simulink model "behav_mcode_ckpt1_2021b_V2"  (R2021b)
settings: Solver=FixedStepDiscrete  StartTime=0.0  StopTime=40  FixedStep=1  RelTol=1e-3
(part 1 of 2)
settings Model: Creator=lisix  LastModifiedBy=lisixu
settings DebuggingCC: UnconnectedInputMsg=none  UnconnectedOutputMsg=none  UnconnectedLineMsg=none
settings RTWCC: DLArmComputeVersion=20.02.1

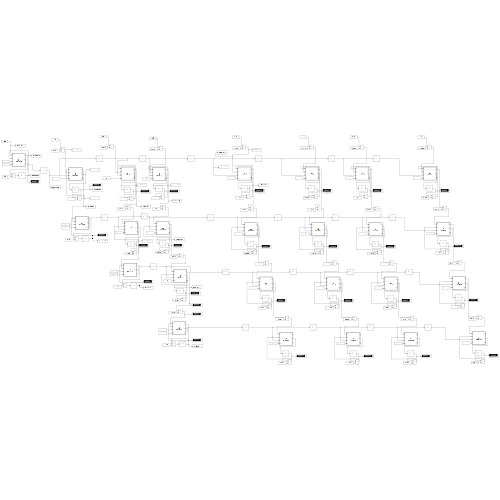
[thumbnail: Simulink's stored preview of the top-level diagram]
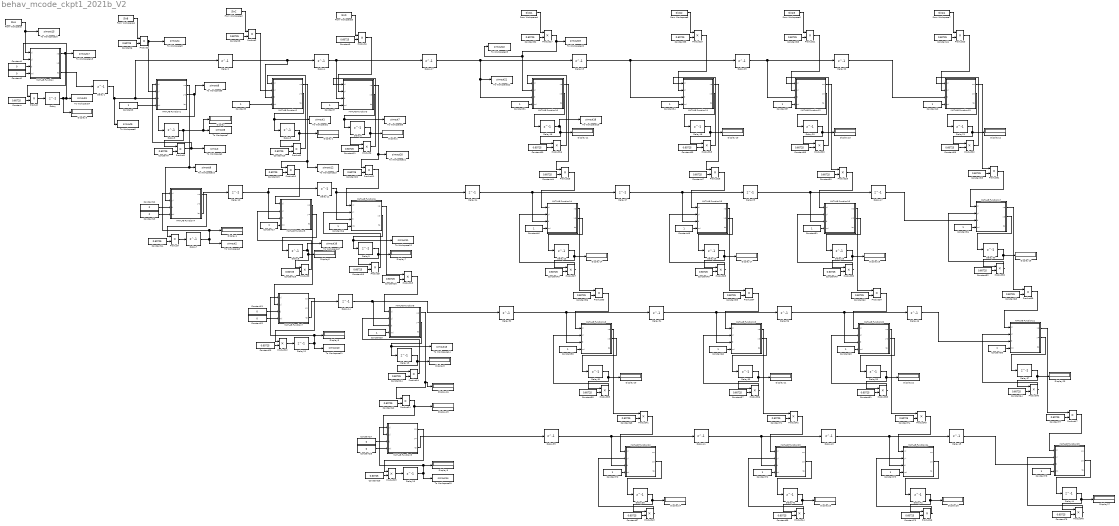
== system behav_mcode_ckpt1_2021b_V2 ==
  Constant{,4,6,8..11,14..15,18..20,23..24,26,29..30,32..33,35..36,38..39,41..45,47,49..50,52..53,55..57,59,61..62,64..65,67..69,71,73..74,76..77} (49 alike) : Constant  Value=0.60725
  Constant{1..2,12..13,21..22,27..28} (8 alike) : Constant  Value=0
  Constant{3,5,7,16..17,25,31,34,37,40,46,48,51,54,58,60,63,66,70,72,75,78} (22 alike) : Constant
  Delay{,1..47} (48 alike) : Delay  DelayLength=1  InitialCondition=0
  Display{,1..27} (28 alike) : Display
  From Workspace : FromWorkspace  VariableName=SlxA  OutputAfterFinalValue=Setting to zero
  From Workspace1 : FromWorkspace  VariableName=SlxB  OutputAfterFinalValue=Setting to zero
  From Workspace2 : FromWorkspace  VariableName=SlxC  OutputAfterFinalValue=Setting to zero
  From Workspace3 : FromWorkspace  VariableName=SlxD  OutputAfterFinalValue=Setting to zero
  From Workspace4 : FromWorkspace  VariableName=SlxQ1  OutputAfterFinalValue=Setting to zero
  From Workspace5 : FromWorkspace  VariableName=SlxQ2  OutputAfterFinalValue=Setting to zero
  From Workspace6 : FromWorkspace  VariableName=SlxQ3  OutputAfterFinalValue=Setting to zero
  From Workspace7 : FromWorkspace  VariableName=SlxQ4  OutputAfterFinalValue=Setting to zero
  MATLAB Function : MATLAB Function  TreatAsAtomicUnit=on
  MATLAB Function1 : MATLAB Function  TreatAsAtomicUnit=on
  MATLAB Function10 : MATLAB Function  TreatAsAtomicUnit=on
  MATLAB Function11 : MATLAB Function  TreatAsAtomicUnit=on
  MATLAB Function12 : MATLAB Function  TreatAsAtomicUnit=on
  MATLAB Function13 : MATLAB Function  TreatAsAtomicUnit=on
  MATLAB Function14 : MATLAB Function  TreatAsAtomicUnit=on
  MATLAB Function15 : MATLAB Function  TreatAsAtomicUnit=on
  MATLAB Function16 : MATLAB Function  TreatAsAtomicUnit=on
  MATLAB Function17 : MATLAB Function  TreatAsAtomicUnit=on
  MATLAB Function18 : MATLAB Function  TreatAsAtomicUnit=on
  MATLAB Function19 : MATLAB Function  TreatAsAtomicUnit=on
  MATLAB Function2 : MATLAB Function  TreatAsAtomicUnit=on
  MATLAB Function20 : MATLAB Function  TreatAsAtomicUnit=on
  MATLAB Function21 : MATLAB Function  TreatAsAtomicUnit=on
  MATLAB Function22 : MATLAB Function  TreatAsAtomicUnit=on
  MATLAB Function23 : MATLAB Function  TreatAsAtomicUnit=on
  MATLAB Function24 : MATLAB Function  TreatAsAtomicUnit=on
  MATLAB Function25 : MATLAB Function  TreatAsAtomicUnit=on
  MATLAB Function3 : MATLAB Function  TreatAsAtomicUnit=on
  MATLAB Function4 : MATLAB Function  TreatAsAtomicUnit=on
  MATLAB Function5 : MATLAB Function  TreatAsAtomicUnit=on
  MATLAB Function6 : MATLAB Function  TreatAsAtomicUnit=on
  MATLAB Function7 : MATLAB Function  TreatAsAtomicUnit=on
  MATLAB Function8 : MATLAB Function  TreatAsAtomicUnit=on
  MATLAB Function9 : MATLAB Function  TreatAsAtomicUnit=on
  Product{,1..48} (49 alike) : Product
  To Workspace1 : ToWorkspace  VariableName=simout1  SaveFormat=Timeseries  SampleTime=-1
  To Workspace10 : ToWorkspace  VariableName=simout9  SaveFormat=Timeseries  SampleTime=-1
  To Workspace11 : ToWorkspace  VariableName=simout10  SaveFormat=Timeseries  SampleTime=-1
  To Workspace12 : ToWorkspace  VariableName=simout11  SaveFormat=Timeseries  SampleTime=-1
  To Workspace13 : ToWorkspace  VariableName=simout12  SaveFormat=Timeseries  SampleTime=-1
  To Workspace14 : ToWorkspace  VariableName=simout13  SaveFormat=Timeseries  SampleTime=-1
  To Workspace15 : ToWorkspace  VariableName=simout14  SaveFormat=Timeseries  SampleTime=-1
  To Workspace16 : ToWorkspace  VariableName=simout15  SaveFormat=Timeseries  SampleTime=-1
  To Workspace17 : ToWorkspace  VariableName=simout16  SaveFormat=Timeseries  SampleTime=-1
  To Workspace18 : ToWorkspace  VariableName=simout17  SaveFormat=Timeseries  SampleTime=-1
  To Workspace19 : ToWorkspace  VariableName=simout18  SaveFormat=Timeseries  SampleTime=-1
  To Workspace2 : ToWorkspace  VariableName=simout  SaveFormat=Timeseries  SampleTime=-1
  To Workspace20 : ToWorkspace  VariableName=simout19  SaveFormat=Timeseries  SampleTime=-1
  To Workspace21 : ToWorkspace  VariableName=simout20  SaveFormat=Timeseries  SampleTime=-1
  To Workspace22 : ToWorkspace  VariableName=simout21  SaveFormat=Timeseries  SampleTime=-1
  To Workspace23 : ToWorkspace  VariableName=simout22  SaveFormat=Timeseries  SampleTime=-1
  To Workspace3 : ToWorkspace  VariableName=simout2  SaveFormat=Timeseries  SampleTime=-1
  To Workspace4 : ToWorkspace  VariableName=simout3  SaveFormat=Timeseries  SampleTime=-1
  To Workspace5 : ToWorkspace  VariableName=simout4  SaveFormat=Timeseries  SampleTime=-1
  To Workspace6 : ToWorkspace  VariableName=simout5  SaveFormat=Timeseries  SampleTime=-1
  To Workspace7 : ToWorkspace  VariableName=simout6  SaveFormat=Timeseries  SampleTime=-1
  To Workspace8 : ToWorkspace  VariableName=simout7  SaveFormat=Timeseries  SampleTime=-1
  To Workspace9 : ToWorkspace  VariableName=simout8  SaveFormat=Timeseries  SampleTime=-1
  wires:
  MATLAB Function/1(xo) -> To Workspace18/1, Product/1
  Product/1 -> Delay/1
  Delay/1 -> Display3/1, MATLAB Function/2(yi), To Workspace4/1
  Constant/1 -> Product/2
  Constant1/1 -> MATLAB Function/3(ti)
  Constant2/1 -> MATLAB Function/4(mi)
  MATLAB Function/3(to) -> Delay1/1
  Constant3/1 -> MATLAB Function1/4(mi)
  Delay1/1 -> To Workspace6/1, Delay2/1, MATLAB Function1/3(ti)
  From Workspace1/1 -> Product3/1
  Delay3/1 -> Display/1, To Workspace7/1, Product1/1
  Constant6/1 -> Product3/2
  Constant4/1 -> Product1/2
  Product1/1 -> MATLAB Function1/1(xi), To Workspace2/1
  Delay2/1 -> Delay4/1, MATLAB Function2/3(ti)
  Constant5/1 -> MATLAB Function2/4(mi)
  Constant7/1 -> MATLAB Function3/4(mi)
  Delay4/1 -> Delay17/1, MATLAB Function3/3(ti)
  Constant8/1 -> Product2/2
  From Workspace2/1 -> Product2/1
  Product2/1 -> MATLAB Function2/2(yi)
  Constant9/1 -> Product4/2
  From Workspace3/1 -> Product4/1
  Product4/1 -> MATLAB Function3/2(yi)
  Constant10/1 -> Product5/2
  Delay5/1 -> Display1/1, Product5/1
  Product5/1 -> MATLAB Function2/1(xi)
  Constant11/1 -> Product6/2
  Delay6/1 -> Display2/1, Product6/1
  Product6/1 -> MATLAB Function3/1(xi)
  Product3/1 -> MATLAB Function1/2(yi), To Workspace5/1
  From Workspace/1 -> To Workspace16/1, MATLAB Function/1(xi)
  MATLAB Function1/2(yo) -> Delay3/1, To Workspace9/1
  MATLAB Function2/2(yo) -> To Workspace1/1, Delay5/1
  MATLAB Function3/2(yo) -> To Workspace8/1, Delay6/1
  Constant12/1 -> MATLAB Function4/3(ti)
  Constant13/1 -> MATLAB Function4/4(mi)
  Constant14/1 -> Product7/2
  Product7/1 -> Delay7/1
  Delay7/1 -> To Workspace3/1, Display4/1, MATLAB Function4/1(xi)
  MATLAB Function4/1(xo) -> Product7/1
  MATLAB Function1/1(xo) -> MATLAB Function4/2(yi), To Workspace10/1
  Constant16/1 -> MATLAB Function6/4(mi)
  Constant15/1 -> Product9/2
  MATLAB Function6/2(yo) -> To Workspace12/1, Delay9/1
  Delay8/1 -> To Workspace17/1, Display6/1, Product8/1
  Delay9/1 -> Display7/1, Product9/1
  MATLAB Function4/3(to) -> Delay10/1
  Delay10/1 -> Delay11/1, MATLAB Function5/3(ti)
  Constant17/1 -> MATLAB Function5/4(mi)
  Delay11/1 -> Delay24/1, MATLAB Function6/3(ti)
  MATLAB Function3/1(xo) -> To Workspace21/1, Product11/1
  Constant18/1 -> Product8/2
  MATLAB Function2/1(xo) -> Product10/1, To Workspace13/1
  Constant19/1 -> Product10/2
  MATLAB Function5/2(yo) -> Delay8/1
  Constant20/1 -> Product11/2
  Product9/1 -> MATLAB Function6/2(yi)
  Product10/1 -> MATLAB Function5/1(xi)
  Product8/1 -> MATLAB Function5/2(yi)
  Constant23/1 -> Product12/2
  Constant21/1 -> MATLAB Function7/3(ti)
  Product12/1 -> Delay12/1
  Delay12/1 -> Display5/1, MATLAB Function7/1(xi), To Workspace11/1
  MATLAB Function7/1(xo) -> Product12/1
  Constant22/1 -> MATLAB Function7/4(mi)
  MATLAB Function5/1(xo) -> MATLAB Function7/2(yi)
  Delay13/1 -> Display8/1, Product14/1
  MATLAB Function8/2(yo) -> To Workspace14/1, Delay13/1
  Constant24/1 -> Product14/2
  Constant25/1 -> MATLAB Function8/4(mi)
  Product14/1 -> MATLAB Function8/2(yi)
  Constant26/1 -> Product13/2
  MATLAB Function6/1(xo) -> Product13/1
  Product13/1 -> MATLAB Function8/1(xi)
  Product11/1 -> MATLAB Function6/1(xi)
  MATLAB Function7/3(to) -> Delay14/1
  MATLAB Function9/1(xo) -> Product15/1
  Constant27/1 -> MATLAB Function9/3(ti)
  Constant28/1 -> MATLAB Function9/4(mi)
  Constant29/1 -> Product15/2
  Product15/1 -> Delay15/1
  Delay15/1 -> Display9/1, MATLAB Function9/1(xi), To Workspace15/1
  Constant31/1 -> MATLAB Function10/4(mi)
  MATLAB Function10/2(yo) -> Delay16/1
  Delay16/1 -> To Workspace19/1, Display11/1, Product16/1
  Constant32/1 -> Product17/2
  From Workspace4/1 -> Product17/1
  Constant30/1 -> Product16/2
  From Workspace5/1 -> Product19/1
  Constant35/1 -> Product19/2
  Product19/1 -> MATLAB Function11/2(yi)
  Constant33/1 -> Product18/2
  Delay18/1 -> Display10/1, Product18/1
  Product18/1 -> MATLAB Function11/1(xi)
  Constant34/1 -> MATLAB Function11/4(mi)
  MATLAB Function11/2(yo) -> Delay18/1
  Delay17/1 -> Delay19/1, To Workspace22/1, MATLAB Function10/3(ti)
  From Workspace6/1 -> Product21/1
  Constant38/1 -> Product21/2
  Product21/1 -> MATLAB Function12/2(yi)
  Constant36/1 -> Product20/2
  Product23/1 -> MATLAB Function13/2(yi)
  Constant41/1 -> Product23/2
  From Workspace7/1 -> Product23/1
  Delay21/1 -> Display12/1, Product22/1
  Constant39/1 -> Product22/2
  Delay20/1 -> Display13/1, Product20/1
  Product20/1 -> MATLAB Function12/1(xi)
  MATLAB Function12/2(yo) -> Delay20/1
  Delay19/1 -> Delay25/1, MATLAB Function11/3(ti)
  MATLAB Function13/2(yo) -> Delay21/1
  Constant40/1 -> MATLAB Function13/4(mi)
  Constant37/1 -> MATLAB Function12/4(mi)
  Product22/1 -> MATLAB Function13/1(xi)
  Constant42/1 -> Product24/2
  Product24/1 -> Display15/1, MATLAB Function9/2(yi)
  Delay24/1 -> Delay27/1, MATLAB Function14/3(ti)
  Delay23/1 -> Display14/1, Product27/1
  MATLAB Function10/1(xo) -> Product25/1
  Constant43/1 -> Product27/2
  Constant46/1 -> MATLAB Function14/4(mi)
  Constant44/1 -> Product25/2
  Delay25/1 -> Delay22/1, MATLAB Function12/3(ti)
  MATLAB Function8/1(xo) -> Product24/1, Display16/1
  Delay22/1 -> MATLAB Function13/3(ti)
  Product27/1 -> MATLAB Function14/2(yi)
  Product25/1 -> MATLAB Function14/1(xi)
  MATLAB Function14/2(yo) -> Delay23/1
  Delay27/1 -> Delay29/1, MATLAB Function15/3(ti)
  Constant47/1 -> Product26/2
  Constant48/1 -> MATLAB Function15/4(mi)
  Constant45/1 -> Product28/2
  MATLAB Function11/1(xo) -> Product26/1
  MATLAB Function15/2(yo) -> Delay26/1
  Product28/1 -> MATLAB Function15/2(yi)
  Delay26/1 -> Display17/1, Product28/1
  Product26/1 -> MATLAB Function15/1(xi)
  MATLAB Function16/2(yo) -> Delay28/1
  Constant49/1 -> Product30/2
  MATLAB Function12/1(xo) -> Product29/1
  Product29/1 -> MATLAB Function16/1(xi)
  Constant51/1 -> MATLAB Function16/4(mi)
  Constant50/1 -> Product29/2
  Delay28/1 -> Display18/1, Product30/1
  Product30/1 -> MATLAB Function16/2(yi)
  Product31/1 -> MATLAB Function17/1(xi)
  Constant53/1 -> Product31/2
  Delay29/1 -> Delay47/1, MATLAB Function16/3(ti)
  Constant54/1 -> MATLAB Function17/4(mi)
  Delay30/1 -> Display19/1, Product32/1
  Constant52/1 -> Product32/2
  MATLAB Function13/1(xo) -> Product31/1
  Product32/1 -> MATLAB Function17/2(yi)
  MATLAB Function17/2(yo) -> Delay30/1
  Delay14/1 -> Delay32/1, MATLAB Function8/3(ti)
  Delay32/1 -> Delay34/1, MATLAB Function18/3(ti)
  MATLAB Function19/2(yo) -> Delay33/1
  Constant56/1 -> Product33/2
  Constant55/1 -> Product35/2
  MATLAB Function15/1(xo) -> Product34/1
  MATLAB Function18/2(yo) -> Delay31/1
  Constant66/1 -> MATLAB Function21/4(mi)
  Delay37/1 -> Display23/1, Product40/1
  Product40/1 -> MATLAB Function21/2(yi)
  Constant64/1 -> Product40/2
  Product34/1 -> MATLAB Function19/1(xi)
  Constant58/1 -> MATLAB Function18/4(mi)
  MATLAB Function21/2(yo) -> Delay37/1
  MATLAB Function14/1(xo) -> Product33/1
  Constant59/1 -> Product34/2
  Delay34/1 -> Delay36/1, MATLAB Function19/3(ti)
  Product33/1 -> MATLAB Function18/1(xi)
  Constant60/1 -> MATLAB Function19/4(mi)
  Delay31/1 -> Display20/1, Product35/1
  MATLAB Function17/1(xo) -> Product39/1
  Product35/1 -> MATLAB Function18/2(yi)
  Product38/1 -> MATLAB Function20/2(yi)
  Constant65/1 -> Product39/2
  Product37/1 -> MATLAB Function20/1(xi)
  Constant62/1 -> Product37/2
  Delay36/1 -> Delay46/1, MATLAB Function20/3(ti)
  Constant57/1 -> Product36/2
  Constant63/1 -> MATLAB Function20/4(mi)
  Constant61/1 -> Product38/2
  MATLAB Function16/1(xo) -> Product37/1
  MATLAB Function20/2(yo) -> Delay35/1
  Product36/1 -> MATLAB Function19/2(yi)
  Product39/1 -> MATLAB Function21/1(xi)
  Delay33/1 -> Display21/1, Product36/1
  Delay35/1 -> Display22/1, Product38/1
  MATLAB Function21/1(xo) -> Product47/1
  MATLAB Function25/2(yo) -> Delay44/1
  Product48/1 -> MATLAB Function25/2(yi)
  Constant78/1 -> MATLAB Function25/4(mi)
  MATLAB Function22/2(yo) -> Delay38/1
  Delay41/1 -> Delay43/1, MATLAB Function23/3(ti)
  Constant67/1 -> Product43/2
  Constant71/1 -> Product42/2
  Constant68/1 -> Product41/2
  MATLAB Function19/1(xo) -> Product42/1
  Constant73/1 -> Product46/2
  Constant69/1 -> Product44/2
  Delay39/1 -> Delay41/1, MATLAB Function22/3(ti)
  Constant75/1 -> MATLAB Function24/4(mi)
  Constant74/1 -> Product45/2
  Delay43/1 -> Delay45/1, MATLAB Function24/3(ti)
  Product42/1 -> MATLAB Function23/1(xi)
  Product43/1 -> MATLAB Function22/2(yi)
  Constant77/1 -> Product47/2
  Product46/1 -> MATLAB Function24/2(yi)
  Product45/1 -> MATLAB Function24/1(xi)
  Delay38/1 -> Display24/1, Product43/1
  Product41/1 -> MATLAB Function22/1(xi)
  MATLAB Function18/1(xo) -> Product41/1
  Constant72/1 -> MATLAB Function23/4(mi)
  Constant76/1 -> Product48/2
  Delay42/1 -> Display26/1, Product46/1
  Delay40/1 -> Display25/1, Product44/1
  Delay44/1 -> Display27/1, Product48/1
  Product44/1 -> MATLAB Function23/2(yi)
  MATLAB Function24/2(yo) -> Delay42/1
  MATLAB Function23/2(yo) -> Delay40/1
  MATLAB Function20/1(xo) -> Product45/1
  Product47/1 -> MATLAB Function25/1(xi)
  Constant70/1 -> MATLAB Function22/4(mi)
  MATLAB Function9/3(to) -> Delay39/1
  Product16/1 -> MATLAB Function10/1(xi)
  Product17/1 -> To Workspace20/1, MATLAB Function10/2(yi), To Workspace23/1
  Delay45/1 -> MATLAB Function25/3(ti)
  Delay46/1 -> MATLAB Function21/3(ti)
  Delay47/1 -> MATLAB Function17/3(ti)

== matlab function behav_mcode_ckpt1_2021b_V2/MATLAB Function8 ==
  data: xi input; xo output; yi input; ti input; mi input; yo output; to output
function [xo,yo,to] = cordicVanilla(xi,yi,ti,mi)
cordic_phase=[0.78539816339744828000,0.46364760900080609000,0.24497866312686414000,0.12435499454676144000,0.06241880999595735000,0.03123983343026827700,0.01562372862047683100,0.00781234106010111110,0.00390623013196697180,0.00195312251647881880,0.00097656218955931946,0.00048828121119489829,0.00024414062014936177,0.00012207031189367021,0.00006103515617420877,0.00003051757811552610,0.00001525878906131576,0.00000762939453110197,0.00000381469726560650,0.00000190734863281019,0.00000095367431640596,0.00000047683715820309,0.00000023841857910156,0.00000011920928955078,0.00000005960464477539,0.00000002980232238770,0.00000001490116119385,0.00000000745058059692,0.00000000372529029846,0.00000000186264514923,0.00000000093132257462,0.00000000046566128731,0.00000000023283064365,0.00000000011641532183,0.00000000005820766091,0.00000000002910383046,0.00000000001455191523,0.00000000000727595761,0.00000000000363797881,0.00000000000181898940,0.00000000000090949470,0.00000000000045474735,0.00000000000022737368,0.00000000000011368684,0.00000000000005684342,0.00000000000002842171,0.00000000000001421085,0.00000000000000710543,0.00000000000000355271,0.00000000000000177636,0.00000000000000088818,0.00000000000000044409,0.00000000000000022204,0.00000000000000011102,0.00000000000000005551,0.00000000000000002776,0.00000000000000001388,0.00000000000000000694,0.00000000000000000347,0.00000000000000000173,0.00000000000000000087,0.00000000000000000043,0.00000000000000000022,0.00000000000000000011];

x = xi;
y = yi;
t = 0;
if mi
    t = ti;
else
    t = 0;
end
for i = 1:1:20
    sigma = 0;
    if mi
        if t < 0
            sigma = -1;
        else
            sigma = 1;
        end
    else
        if y < 0
            sigma = 1;
        else
            sigma = -1;
        end
    end
    xs = x * sigma * 2^(-(i-1));
    ys = y * sigma * 2^(-(i-1));
    x = x - ys;
    y = y + xs;
    t = t - sigma * cordic_phase(i);
end
xo = x;
yo = y;
to = t;
end

== matlab function behav_mcode_ckpt1_2021b_V2/MATLAB Function1 ==
  data: xi input; xo output; yi input; ti input; mi input; yo output; to output
function [xo,yo,to] = cordicVanilla(xi,yi,ti,mi)
cordic_phase=[0.78539816339744828000,0.46364760900080609000,0.24497866312686414000,0.12435499454676144000,0.06241880999595735000,0.03123983343026827700,0.01562372862047683100,0.00781234106010111110,0.00390623013196697180,0.00195312251647881880,0.00097656218955931946,0.00048828121119489829,0.00024414062014936177,0.00012207031189367021,0.00006103515617420877,0.00003051757811552610,0.00001525878906131576,0.00000762939453110197,0.00000381469726560650,0.00000190734863281019,0.00000095367431640596,0.00000047683715820309,0.00000023841857910156,0.00000011920928955078,0.00000005960464477539,0.00000002980232238770,0.00000001490116119385,0.00000000745058059692,0.00000000372529029846,0.00000000186264514923,0.00000000093132257462,0.00000000046566128731,0.00000000023283064365,0.00000000011641532183,0.00000000005820766091,0.00000000002910383046,0.00000000001455191523,0.00000000000727595761,0.00000000000363797881,0.00000000000181898940,0.00000000000090949470,0.00000000000045474735,0.00000000000022737368,0.00000000000011368684,0.00000000000005684342,0.00000000000002842171,0.00000000000001421085,0.00000000000000710543,0.00000000000000355271,0.00000000000000177636,0.00000000000000088818,0.00000000000000044409,0.00000000000000022204,0.00000000000000011102,0.00000000000000005551,0.00000000000000002776,0.00000000000000001388,0.00000000000000000694,0.00000000000000000347,0.00000000000000000173,0.00000000000000000087,0.00000000000000000043,0.00000000000000000022,0.00000000000000000011];

x = xi;
y = yi;
t = 0;
if mi
    t = ti;
else
    t = 0;
end
for i = 1:1:10
    sigma = 0;
    if mi
        if t < 0
            sigma = -1;
        else
            sigma = 1;
        end
    else
        if y < 0
            sigma = 1;
        else
            sigma = -1;
        end
    end
    xs = x * sigma * 2^(-(i-1));
    ys = y * sigma * 2^(-(i-1));
    x = x - ys;
    y = y + xs;
    t = t - sigma * cordic_phase(i);
end
xo = x;
yo = y;
to = t;
end

== matlab function behav_mcode_ckpt1_2021b_V2/MATLAB Function9 ==
  data: xi input; xo output; yi input; ti input; mi input; yo output; to output
function [xo,yo,to] = cordicVanilla(xi,yi,ti,mi)
cordic_phase=[0.78539816339744828000,0.46364760900080609000,0.24497866312686414000,0.12435499454676144000,0.06241880999595735000,0.03123983343026827700,0.01562372862047683100,0.00781234106010111110,0.00390623013196697180,0.00195312251647881880,0.00097656218955931946,0.00048828121119489829,0.00024414062014936177,0.00012207031189367021,0.00006103515617420877,0.00003051757811552610,0.00001525878906131576,0.00000762939453110197,0.00000381469726560650,0.00000190734863281019,0.00000095367431640596,0.00000047683715820309,0.00000023841857910156,0.00000011920928955078,0.00000005960464477539,0.00000002980232238770,0.00000001490116119385,0.00000000745058059692,0.00000000372529029846,0.00000000186264514923,0.00000000093132257462,0.00000000046566128731,0.00000000023283064365,0.00000000011641532183,0.00000000005820766091,0.00000000002910383046,0.00000000001455191523,0.00000000000727595761,0.00000000000363797881,0.00000000000181898940,0.00000000000090949470,0.00000000000045474735,0.00000000000022737368,0.00000000000011368684,0.00000000000005684342,0.00000000000002842171,0.00000000000001421085,0.00000000000000710543,0.00000000000000355271,0.00000000000000177636,0.00000000000000088818,0.00000000000000044409,0.00000000000000022204,0.00000000000000011102,0.00000000000000005551,0.00000000000000002776,0.00000000000000001388,0.00000000000000000694,0.00000000000000000347,0.00000000000000000173,0.00000000000000000087,0.00000000000000000043,0.00000000000000000022,0.00000000000000000011];

x = xi;
y = yi;
t = 0;
if mi
    t = ti;
else
    t = 0;
end
for i = 1:1:10
    sigma = 0;
    if mi
        if t < 0
            sigma = -1;
        else
            sigma = 1;
        end
    else
        if y < 0
            sigma = 1;
        else
            sigma = -1;
        end
    end
    xs = x * sigma * 2^(-(i-1));
    ys = y * sigma * 2^(-(i-1));
    x = x - ys;
    y = y + xs;
    t = t - sigma * cordic_phase(i);
end
xo = x;
yo = y;
to = t;
end

== matlab function behav_mcode_ckpt1_2021b_V2/MATLAB Function10 ==
  data: xi input; xo output; yi input; ti input; mi input; yo output; to output
function [xo,yo,to] = cordicVanilla(xi,yi,ti,mi)
cordic_phase=[0.78539816339744828000,0.46364760900080609000,0.24497866312686414000,0.12435499454676144000,0.06241880999595735000,0.03123983343026827700,0.01562372862047683100,0.00781234106010111110,0.00390623013196697180,0.00195312251647881880,0.00097656218955931946,0.00048828121119489829,0.00024414062014936177,0.00012207031189367021,0.00006103515617420877,0.00003051757811552610,0.00001525878906131576,0.00000762939453110197,0.00000381469726560650,0.00000190734863281019,0.00000095367431640596,0.00000047683715820309,0.00000023841857910156,0.00000011920928955078,0.00000005960464477539,0.00000002980232238770,0.00000001490116119385,0.00000000745058059692,0.00000000372529029846,0.00000000186264514923,0.00000000093132257462,0.00000000046566128731,0.00000000023283064365,0.00000000011641532183,0.00000000005820766091,0.00000000002910383046,0.00000000001455191523,0.00000000000727595761,0.00000000000363797881,0.00000000000181898940,0.00000000000090949470,0.00000000000045474735,0.00000000000022737368,0.00000000000011368684,0.00000000000005684342,0.00000000000002842171,0.00000000000001421085,0.00000000000000710543,0.00000000000000355271,0.00000000000000177636,0.00000000000000088818,0.00000000000000044409,0.00000000000000022204,0.00000000000000011102,0.00000000000000005551,0.00000000000000002776,0.00000000000000001388,0.00000000000000000694,0.00000000000000000347,0.00000000000000000173,0.00000000000000000087,0.00000000000000000043,0.00000000000000000022,0.00000000000000000011];

x = xi;
y = yi;
t = 0;
if mi
    t = ti;
else
    t = 0;
end
for i = 1:1:20
    sigma = 0;
    if mi
        if t < 0
            sigma = -1;
        else
            sigma = 1;
        end
    else
        if y < 0
            sigma = 1;
        else
            sigma = -1;
        end
    end
    xs = x * sigma * 2^(-(i-1));
    ys = y * sigma * 2^(-(i-1));
    x = x - ys;
    y = y + xs;
    t = t - sigma * cordic_phase(i);
end
xo = x;
yo = y;
to = t;
end

== matlab function behav_mcode_ckpt1_2021b_V2/MATLAB Function11 ==
  data: xi input; xo output; yi input; ti input; mi input; yo output; to output
function [xo,yo,to] = cordicVanilla(xi,yi,ti,mi)
cordic_phase=[0.78539816339744828000,0.46364760900080609000,0.24497866312686414000,0.12435499454676144000,0.06241880999595735000,0.03123983343026827700,0.01562372862047683100,0.00781234106010111110,0.00390623013196697180,0.00195312251647881880,0.00097656218955931946,0.00048828121119489829,0.00024414062014936177,0.00012207031189367021,0.00006103515617420877,0.00003051757811552610,0.00001525878906131576,0.00000762939453110197,0.00000381469726560650,0.00000190734863281019,0.00000095367431640596,0.00000047683715820309,0.00000023841857910156,0.00000011920928955078,0.00000005960464477539,0.00000002980232238770,0.00000001490116119385,0.00000000745058059692,0.00000000372529029846,0.00000000186264514923,0.00000000093132257462,0.00000000046566128731,0.00000000023283064365,0.00000000011641532183,0.00000000005820766091,0.00000000002910383046,0.00000000001455191523,0.00000000000727595761,0.00000000000363797881,0.00000000000181898940,0.00000000000090949470,0.00000000000045474735,0.00000000000022737368,0.00000000000011368684,0.00000000000005684342,0.00000000000002842171,0.00000000000001421085,0.00000000000000710543,0.00000000000000355271,0.00000000000000177636,0.00000000000000088818,0.00000000000000044409,0.00000000000000022204,0.00000000000000011102,0.00000000000000005551,0.00000000000000002776,0.00000000000000001388,0.00000000000000000694,0.00000000000000000347,0.00000000000000000173,0.00000000000000000087,0.00000000000000000043,0.00000000000000000022,0.00000000000000000011];

x = xi;
y = yi;
t = 0;
if mi
    t = ti;
else
    t = 0;
end
for i = 1:1:30
    sigma = 0;
    if mi
        if t < 0
            sigma = -1;
        else
            sigma = 1;
        end
    else
        if y < 0
            sigma = 1;
        else
            sigma = -1;
        end
    end
    xs = x * sigma * 2^(-(i-1));
    ys = y * sigma * 2^(-(i-1));
    x = x - ys;
    y = y + xs;
    t = t - sigma * cordic_phase(i);
end
xo = x;
yo = y;
to = t;
end

== matlab function behav_mcode_ckpt1_2021b_V2/MATLAB Function12 ==
  data: xi input; xo output; yi input; ti input; mi input; yo output; to output
function [xo,yo,to] = cordicVanilla(xi,yi,ti,mi)
cordic_phase=[0.78539816339744828000,0.46364760900080609000,0.24497866312686414000,0.12435499454676144000,0.06241880999595735000,0.03123983343026827700,0.01562372862047683100,0.00781234106010111110,0.00390623013196697180,0.00195312251647881880,0.00097656218955931946,0.00048828121119489829,0.00024414062014936177,0.00012207031189367021,0.00006103515617420877,0.00003051757811552610,0.00001525878906131576,0.00000762939453110197,0.00000381469726560650,0.00000190734863281019,0.00000095367431640596,0.00000047683715820309,0.00000023841857910156,0.00000011920928955078,0.00000005960464477539,0.00000002980232238770,0.00000001490116119385,0.00000000745058059692,0.00000000372529029846,0.00000000186264514923,0.00000000093132257462,0.00000000046566128731,0.00000000023283064365,0.00000000011641532183,0.00000000005820766091,0.00000000002910383046,0.00000000001455191523,0.00000000000727595761,0.00000000000363797881,0.00000000000181898940,0.00000000000090949470,0.00000000000045474735,0.00000000000022737368,0.00000000000011368684,0.00000000000005684342,0.00000000000002842171,0.00000000000001421085,0.00000000000000710543,0.00000000000000355271,0.00000000000000177636,0.00000000000000088818,0.00000000000000044409,0.00000000000000022204,0.00000000000000011102,0.00000000000000005551,0.00000000000000002776,0.00000000000000001388,0.00000000000000000694,0.00000000000000000347,0.00000000000000000173,0.00000000000000000087,0.00000000000000000043,0.00000000000000000022,0.00000000000000000011];

x = xi;
y = yi;
t = 0;
if mi
    t = ti;
else
    t = 0;
end
for i = 1:1:20
    sigma = 0;
    if mi
        if t < 0
            sigma = -1;
        else
            sigma = 1;
        end
    else
        if y < 0
            sigma = 1;
        else
            sigma = -1;
        end
    end
    xs = x * sigma * 2^(-(i-1));
    ys = y * sigma * 2^(-(i-1));
    x = x - ys;
    y = y + xs;
    t = t - sigma * cordic_phase(i);
end
xo = x;
yo = y;
to = t;
end

== matlab function behav_mcode_ckpt1_2021b_V2/MATLAB Function13 ==
  data: xi input; xo output; yi input; ti input; mi input; yo output; to output
function [xo,yo,to] = cordicVanilla(xi,yi,ti,mi)
cordic_phase=[0.78539816339744828000,0.46364760900080609000,0.24497866312686414000,0.12435499454676144000,0.06241880999595735000,0.03123983343026827700,0.01562372862047683100,0.00781234106010111110,0.00390623013196697180,0.00195312251647881880,0.00097656218955931946,0.00048828121119489829,0.00024414062014936177,0.00012207031189367021,0.00006103515617420877,0.00003051757811552610,0.00001525878906131576,0.00000762939453110197,0.00000381469726560650,0.00000190734863281019,0.00000095367431640596,0.00000047683715820309,0.00000023841857910156,0.00000011920928955078,0.00000005960464477539,0.00000002980232238770,0.00000001490116119385,0.00000000745058059692,0.00000000372529029846,0.00000000186264514923,0.00000000093132257462,0.00000000046566128731,0.00000000023283064365,0.00000000011641532183,0.00000000005820766091,0.00000000002910383046,0.00000000001455191523,0.00000000000727595761,0.00000000000363797881,0.00000000000181898940,0.00000000000090949470,0.00000000000045474735,0.00000000000022737368,0.00000000000011368684,0.00000000000005684342,0.00000000000002842171,0.00000000000001421085,0.00000000000000710543,0.00000000000000355271,0.00000000000000177636,0.00000000000000088818,0.00000000000000044409,0.00000000000000022204,0.00000000000000011102,0.00000000000000005551,0.00000000000000002776,0.00000000000000001388,0.00000000000000000694,0.00000000000000000347,0.00000000000000000173,0.00000000000000000087,0.00000000000000000043,0.00000000000000000022,0.00000000000000000011];

x = xi;
y = yi;
t = 0;
if mi
    t = ti;
else
    t = 0;
end
for i = 1:1:20
    sigma = 0;
    if mi
        if t < 0
            sigma = -1;
        else
            sigma = 1;
        end
    else
        if y < 0
            sigma = 1;
        else
            sigma = -1;
        end
    end
    xs = x * sigma * 2^(-(i-1));
    ys = y * sigma * 2^(-(i-1));
    x = x - ys;
    y = y + xs;
    t = t - sigma * cordic_phase(i);
end
xo = x;
yo = y;
to = t;
end

== matlab function behav_mcode_ckpt1_2021b_V2/MATLAB Function14 ==
  data: xi input; xo output; yi input; ti input; mi input; yo output; to output
function [xo,yo,to] = cordicVanilla(xi,yi,ti,mi)
cordic_phase=[0.78539816339744828000,0.46364760900080609000,0.24497866312686414000,0.12435499454676144000,0.06241880999595735000,0.03123983343026827700,0.01562372862047683100,0.00781234106010111110,0.00390623013196697180,0.00195312251647881880,0.00097656218955931946,0.00048828121119489829,0.00024414062014936177,0.00012207031189367021,0.00006103515617420877,0.00003051757811552610,0.00001525878906131576,0.00000762939453110197,0.00000381469726560650,0.00000190734863281019,0.00000095367431640596,0.00000047683715820309,0.00000023841857910156,0.00000011920928955078,0.00000005960464477539,0.00000002980232238770,0.00000001490116119385,0.00000000745058059692,0.00000000372529029846,0.00000000186264514923,0.00000000093132257462,0.00000000046566128731,0.00000000023283064365,0.00000000011641532183,0.00000000005820766091,0.00000000002910383046,0.00000000001455191523,0.00000000000727595761,0.00000000000363797881,0.00000000000181898940,0.00000000000090949470,0.00000000000045474735,0.00000000000022737368,0.00000000000011368684,0.00000000000005684342,0.00000000000002842171,0.00000000000001421085,0.00000000000000710543,0.00000000000000355271,0.00000000000000177636,0.00000000000000088818,0.00000000000000044409,0.00000000000000022204,0.00000000000000011102,0.00000000000000005551,0.00000000000000002776,0.00000000000000001388,0.00000000000000000694,0.00000000000000000347,0.00000000000000000173,0.00000000000000000087,0.00000000000000000043,0.00000000000000000022,0.00000000000000000011];

x = xi;
y = yi;
t = 0;
if mi
    t = ti;
else
    t = 0;
end
for i = 1:1:20
    sigma = 0;
    if mi
        if t < 0
            sigma = -1;
        else
            sigma = 1;
        end
    else
        if y < 0
            sigma = 1;
        else
            sigma = -1;
        end
    end
    xs = x * sigma * 2^(-(i-1));
    ys = y * sigma * 2^(-(i-1));
    x = x - ys;
    y = y + xs;
    t = t - sigma * cordic_phase(i);
end
xo = x;
yo = y;
to = t;
end

== matlab function behav_mcode_ckpt1_2021b_V2/MATLAB Function15 ==
  data: xi input; xo output; yi input; ti input; mi input; yo output; to output
function [xo,yo,to] = cordicVanilla(xi,yi,ti,mi)
cordic_phase=[0.78539816339744828000,0.46364760900080609000,0.24497866312686414000,0.12435499454676144000,0.06241880999595735000,0.03123983343026827700,0.01562372862047683100,0.00781234106010111110,0.00390623013196697180,0.00195312251647881880,0.00097656218955931946,0.00048828121119489829,0.00024414062014936177,0.00012207031189367021,0.00006103515617420877,0.00003051757811552610,0.00001525878906131576,0.00000762939453110197,0.00000381469726560650,0.00000190734863281019,0.00000095367431640596,0.00000047683715820309,0.00000023841857910156,0.00000011920928955078,0.00000005960464477539,0.00000002980232238770,0.00000001490116119385,0.00000000745058059692,0.00000000372529029846,0.00000000186264514923,0.00000000093132257462,0.00000000046566128731,0.00000000023283064365,0.00000000011641532183,0.00000000005820766091,0.00000000002910383046,0.00000000001455191523,0.00000000000727595761,0.00000000000363797881,0.00000000000181898940,0.00000000000090949470,0.00000000000045474735,0.00000000000022737368,0.00000000000011368684,0.00000000000005684342,0.00000000000002842171,0.00000000000001421085,0.00000000000000710543,0.00000000000000355271,0.00000000000000177636,0.00000000000000088818,0.00000000000000044409,0.00000000000000022204,0.00000000000000011102,0.00000000000000005551,0.00000000000000002776,0.00000000000000001388,0.00000000000000000694,0.00000000000000000347,0.00000000000000000173,0.00000000000000000087,0.00000000000000000043,0.00000000000000000022,0.00000000000000000011];

x = xi;
y = yi;
t = 0;
if mi
    t = ti;
else
    t = 0;
end
for i = 1:1:20
    sigma = 0;
    if mi
        if t < 0
            sigma = -1;
        else
            sigma = 1;
        end
    else
        if y < 0
            sigma = 1;
        else
            sigma = -1;
        end
    end
    xs = x * sigma * 2^(-(i-1));
    ys = y * sigma * 2^(-(i-1));
    x = x - ys;
    y = y + xs;
    t = t - sigma * cordic_phase(i);
end
xo = x;
yo = y;
to = t;
end

== matlab function behav_mcode_ckpt1_2021b_V2/MATLAB Function16 ==
  data: xi input; xo output; yi input; ti input; mi input; yo output; to output
function [xo,yo,to] = cordicVanilla(xi,yi,ti,mi)
cordic_phase=[0.78539816339744828000,0.46364760900080609000,0.24497866312686414000,0.12435499454676144000,0.06241880999595735000,0.03123983343026827700,0.01562372862047683100,0.00781234106010111110,0.00390623013196697180,0.00195312251647881880,0.00097656218955931946,0.00048828121119489829,0.00024414062014936177,0.00012207031189367021,0.00006103515617420877,0.00003051757811552610,0.00001525878906131576,0.00000762939453110197,0.00000381469726560650,0.00000190734863281019,0.00000095367431640596,0.00000047683715820309,0.00000023841857910156,0.00000011920928955078,0.00000005960464477539,0.00000002980232238770,0.00000001490116119385,0.00000000745058059692,0.00000000372529029846,0.00000000186264514923,0.00000000093132257462,0.00000000046566128731,0.00000000023283064365,0.00000000011641532183,0.00000000005820766091,0.00000000002910383046,0.00000000001455191523,0.00000000000727595761,0.00000000000363797881,0.00000000000181898940,0.00000000000090949470,0.00000000000045474735,0.00000000000022737368,0.00000000000011368684,0.00000000000005684342,0.00000000000002842171,0.00000000000001421085,0.00000000000000710543,0.00000000000000355271,0.00000000000000177636,0.00000000000000088818,0.00000000000000044409,0.00000000000000022204,0.00000000000000011102,0.00000000000000005551,0.00000000000000002776,0.00000000000000001388,0.00000000000000000694,0.00000000000000000347,0.00000000000000000173,0.00000000000000000087,0.00000000000000000043,0.00000000000000000022,0.00000000000000000011];

x = xi;
y = yi;
t = 0;
if mi
    t = ti;
else
    t = 0;
end
for i = 1:1:20
    sigma = 0;
    if mi
        if t < 0
            sigma = -1;
        else
            sigma = 1;
        end
    else
        if y < 0
            sigma = 1;
        else
            sigma = -1;
        end
    end
    xs = x * sigma * 2^(-(i-1));
    ys = y * sigma * 2^(-(i-1));
    x = x - ys;
    y = y + xs;
    t = t - sigma * cordic_phase(i);
end
xo = x;
yo = y;
to = t;
end

== matlab function behav_mcode_ckpt1_2021b_V2/MATLAB Function17 ==
  data: xi input; xo output; yi input; ti input; mi input; yo output; to output
function [xo,yo,to] = cordicVanilla(xi,yi,ti,mi)
cordic_phase=[0.78539816339744828000,0.46364760900080609000,0.24497866312686414000,0.12435499454676144000,0.06241880999595735000,0.03123983343026827700,0.01562372862047683100,0.00781234106010111110,0.00390623013196697180,0.00195312251647881880,0.00097656218955931946,0.00048828121119489829,0.00024414062014936177,0.00012207031189367021,0.00006103515617420877,0.00003051757811552610,0.00001525878906131576,0.00000762939453110197,0.00000381469726560650,0.00000190734863281019,0.00000095367431640596,0.00000047683715820309,0.00000023841857910156,0.00000011920928955078,0.00000005960464477539,0.00000002980232238770,0.00000001490116119385,0.00000000745058059692,0.00000000372529029846,0.00000000186264514923,0.00000000093132257462,0.00000000046566128731,0.00000000023283064365,0.00000000011641532183,0.00000000005820766091,0.00000000002910383046,0.00000000001455191523,0.00000000000727595761,0.00000000000363797881,0.00000000000181898940,0.00000000000090949470,0.00000000000045474735,0.00000000000022737368,0.00000000000011368684,0.00000000000005684342,0.00000000000002842171,0.00000000000001421085,0.00000000000000710543,0.00000000000000355271,0.00000000000000177636,0.00000000000000088818,0.00000000000000044409,0.00000000000000022204,0.00000000000000011102,0.00000000000000005551,0.00000000000000002776,0.00000000000000001388,0.00000000000000000694,0.00000000000000000347,0.00000000000000000173,0.00000000000000000087,0.00000000000000000043,0.00000000000000000022,0.00000000000000000011];

x = xi;
y = yi;
t = 0;
if mi
    t = ti;
else
    t = 0;
end
for i = 1:1:20
    sigma = 0;
    if mi
        if t < 0
            sigma = -1;
        else
            sigma = 1;
        end
    else
        if y < 0
            sigma = 1;
        else
            sigma = -1;
        end
    end
    xs = x * sigma * 2^(-(i-1));
    ys = y * sigma * 2^(-(i-1));
    x = x - ys;
    y = y + xs;
    t = t - sigma * cordic_phase(i);
end
xo = x;
yo = y;
to = t;
end

== matlab function behav_mcode_ckpt1_2021b_V2/MATLAB Function18 ==
  data: xi input; xo output; yi input; ti input; mi input; yo output; to output
function [xo,yo,to] = cordicVanilla(xi,yi,ti,mi)
cordic_phase=[0.78539816339744828000,0.46364760900080609000,0.24497866312686414000,0.12435499454676144000,0.06241880999595735000,0.03123983343026827700,0.01562372862047683100,0.00781234106010111110,0.00390623013196697180,0.00195312251647881880,0.00097656218955931946,0.00048828121119489829,0.00024414062014936177,0.00012207031189367021,0.00006103515617420877,0.00003051757811552610,0.00001525878906131576,0.00000762939453110197,0.00000381469726560650,0.00000190734863281019,0.00000095367431640596,0.00000047683715820309,0.00000023841857910156,0.00000011920928955078,0.00000005960464477539,0.00000002980232238770,0.00000001490116119385,0.00000000745058059692,0.00000000372529029846,0.00000000186264514923,0.00000000093132257462,0.00000000046566128731,0.00000000023283064365,0.00000000011641532183,0.00000000005820766091,0.00000000002910383046,0.00000000001455191523,0.00000000000727595761,0.00000000000363797881,0.00000000000181898940,0.00000000000090949470,0.00000000000045474735,0.00000000000022737368,0.00000000000011368684,0.00000000000005684342,0.00000000000002842171,0.00000000000001421085,0.00000000000000710543,0.00000000000000355271,0.00000000000000177636,0.00000000000000088818,0.00000000000000044409,0.00000000000000022204,0.00000000000000011102,0.00000000000000005551,0.00000000000000002776,0.00000000000000001388,0.00000000000000000694,0.00000000000000000347,0.00000000000000000173,0.00000000000000000087,0.00000000000000000043,0.00000000000000000022,0.00000000000000000011];

x = xi;
y = yi;
t = 0;
if mi
    t = ti;
else
    t = 0;
end
for i = 1:1:20
    sigma = 0;
    if mi
        if t < 0
            sigma = -1;
        else
            sigma = 1;
        end
    else
        if y < 0
            sigma = 1;
        else
            sigma = -1;
        end
    end
    xs = x * sigma * 2^(-(i-1));
    ys = y * sigma * 2^(-(i-1));
    x = x - ys;
    y = y + xs;
    t = t - sigma * cordic_phase(i);
end
xo = x;
yo = y;
to = t;
end

== matlab function behav_mcode_ckpt1_2021b_V2/MATLAB Function ==
  data: xi input; xo output; yi input; ti input; mi input; yo output; to output
function [xo,yo,to] = cordicVanilla(xi,yi,ti,mi)
cordic_phase=[0.78539816339744828000,0.46364760900080609000,0.24497866312686414000,0.12435499454676144000,0.06241880999595735000,0.03123983343026827700,0.01562372862047683100,0.00781234106010111110,0.00390623013196697180,0.00195312251647881880,0.00097656218955931946,0.00048828121119489829,0.00024414062014936177,0.00012207031189367021,0.00006103515617420877,0.00003051757811552610,0.00001525878906131576,0.00000762939453110197,0.00000381469726560650,0.00000190734863281019,0.00000095367431640596,0.00000047683715820309,0.00000023841857910156,0.00000011920928955078,0.00000005960464477539,0.00000002980232238770,0.00000001490116119385,0.00000000745058059692,0.00000000372529029846,0.00000000186264514923,0.00000000093132257462,0.00000000046566128731,0.00000000023283064365,0.00000000011641532183,0.00000000005820766091,0.00000000002910383046,0.00000000001455191523,0.00000000000727595761,0.00000000000363797881,0.00000000000181898940,0.00000000000090949470,0.00000000000045474735,0.00000000000022737368,0.00000000000011368684,0.00000000000005684342,0.00000000000002842171,0.00000000000001421085,0.00000000000000710543,0.00000000000000355271,0.00000000000000177636,0.00000000000000088818,0.00000000000000044409,0.00000000000000022204,0.00000000000000011102,0.00000000000000005551,0.00000000000000002776,0.00000000000000001388,0.00000000000000000694,0.00000000000000000347,0.00000000000000000173,0.00000000000000000087,0.00000000000000000043,0.00000000000000000022,0.00000000000000000011];

x = xi;
y = yi;
t = 0;
if mi
    t = ti;
else
    t = 0;
end
for i = 1:1:10
    sigma = 0;
    if mi
        if t < 0
            sigma = -1;
        else
            sigma = 1;
        end
    else
        if y < 0
            sigma = 1;
        else
            sigma = -1;
        end
    end
    xs = x * sigma * 2^(-(i-1));
    ys = y * sigma * 2^(-(i-1));
    x = x - ys;
    y = y + xs;
    t = t - sigma * cordic_phase(i);
end
xo = x;
yo = y;
to = t;
end

== matlab function behav_mcode_ckpt1_2021b_V2/MATLAB Function19 ==
  data: xi input; xo output; yi input; ti input; mi input; yo output; to output
function [xo,yo,to] = cordicVanilla(xi,yi,ti,mi)
cordic_phase=[0.78539816339744828000,0.46364760900080609000,0.24497866312686414000,0.12435499454676144000,0.06241880999595735000,0.03123983343026827700,0.01562372862047683100,0.00781234106010111110,0.00390623013196697180,0.00195312251647881880,0.00097656218955931946,0.00048828121119489829,0.00024414062014936177,0.00012207031189367021,0.00006103515617420877,0.00003051757811552610,0.00001525878906131576,0.00000762939453110197,0.00000381469726560650,0.00000190734863281019,0.00000095367431640596,0.00000047683715820309,0.00000023841857910156,0.00000011920928955078,0.00000005960464477539,0.00000002980232238770,0.00000001490116119385,0.00000000745058059692,0.00000000372529029846,0.00000000186264514923,0.00000000093132257462,0.00000000046566128731,0.00000000023283064365,0.00000000011641532183,0.00000000005820766091,0.00000000002910383046,0.00000000001455191523,0.00000000000727595761,0.00000000000363797881,0.00000000000181898940,0.00000000000090949470,0.00000000000045474735,0.00000000000022737368,0.00000000000011368684,0.00000000000005684342,0.00000000000002842171,0.00000000000001421085,0.00000000000000710543,0.00000000000000355271,0.00000000000000177636,0.00000000000000088818,0.00000000000000044409,0.00000000000000022204,0.00000000000000011102,0.00000000000000005551,0.00000000000000002776,0.00000000000000001388,0.00000000000000000694,0.00000000000000000347,0.00000000000000000173,0.00000000000000000087,0.00000000000000000043,0.00000000000000000022,0.00000000000000000011];

x = xi;
y = yi;
t = 0;
if mi
    t = ti;
else
    t = 0;
end
for i = 1:1:20
    sigma = 0;
    if mi
        if t < 0
            sigma = -1;
        else
            sigma = 1;
        end
    else
        if y < 0
            sigma = 1;
        else
            sigma = -1;
        end
    end
    xs = x * sigma * 2^(-(i-1));
    ys = y * sigma * 2^(-(i-1));
    x = x - ys;
    y = y + xs;
    t = t - sigma * cordic_phase(i);
end
xo = x;
yo = y;
to = t;
end

== matlab function behav_mcode_ckpt1_2021b_V2/MATLAB Function20 ==
  data: xi input; xo output; yi input; ti input; mi input; yo output; to output
function [xo,yo,to] = cordicVanilla(xi,yi,ti,mi)
cordic_phase=[0.78539816339744828000,0.46364760900080609000,0.24497866312686414000,0.12435499454676144000,0.06241880999595735000,0.03123983343026827700,0.01562372862047683100,0.00781234106010111110,0.00390623013196697180,0.00195312251647881880,0.00097656218955931946,0.00048828121119489829,0.00024414062014936177,0.00012207031189367021,0.00006103515617420877,0.00003051757811552610,0.00001525878906131576,0.00000762939453110197,0.00000381469726560650,0.00000190734863281019,0.00000095367431640596,0.00000047683715820309,0.00000023841857910156,0.00000011920928955078,0.00000005960464477539,0.00000002980232238770,0.00000001490116119385,0.00000000745058059692,0.00000000372529029846,0.00000000186264514923,0.00000000093132257462,0.00000000046566128731,0.00000000023283064365,0.00000000011641532183,0.00000000005820766091,0.00000000002910383046,0.00000000001455191523,0.00000000000727595761,0.00000000000363797881,0.00000000000181898940,0.00000000000090949470,0.00000000000045474735,0.00000000000022737368,0.00000000000011368684,0.00000000000005684342,0.00000000000002842171,0.00000000000001421085,0.00000000000000710543,0.00000000000000355271,0.00000000000000177636,0.00000000000000088818,0.00000000000000044409,0.00000000000000022204,0.00000000000000011102,0.00000000000000005551,0.00000000000000002776,0.00000000000000001388,0.00000000000000000694,0.00000000000000000347,0.00000000000000000173,0.00000000000000000087,0.00000000000000000043,0.00000000000000000022,0.00000000000000000011];

x = xi;
y = yi;
t = 0;
if mi
    t = ti;
else
    t = 0;
end
for i = 1:1:20
    sigma = 0;
    if mi
        if t < 0
            sigma = -1;
        else
            sigma = 1;
        end
    else
        if y < 0
            sigma = 1;
        else
            sigma = -1;
        end
    end
    xs = x * sigma * 2^(-(i-1));
    ys = y * sigma * 2^(-(i-1));
    x = x - ys;
    y = y + xs;
    t = t - sigma * cordic_phase(i);
end
xo = x;
yo = y;
to = t;
end

== matlab function behav_mcode_ckpt1_2021b_V2/MATLAB Function21 ==
  data: xi input; xo output; yi input; ti input; mi input; yo output; to output
function [xo,yo,to] = cordicVanilla(xi,yi,ti,mi)
cordic_phase=[0.78539816339744828000,0.46364760900080609000,0.24497866312686414000,0.12435499454676144000,0.06241880999595735000,0.03123983343026827700,0.01562372862047683100,0.00781234106010111110,0.00390623013196697180,0.00195312251647881880,0.00097656218955931946,0.00048828121119489829,0.00024414062014936177,0.00012207031189367021,0.00006103515617420877,0.00003051757811552610,0.00001525878906131576,0.00000762939453110197,0.00000381469726560650,0.00000190734863281019,0.00000095367431640596,0.00000047683715820309,0.00000023841857910156,0.00000011920928955078,0.00000005960464477539,0.00000002980232238770,0.00000001490116119385,0.00000000745058059692,0.00000000372529029846,0.00000000186264514923,0.00000000093132257462,0.00000000046566128731,0.00000000023283064365,0.00000000011641532183,0.00000000005820766091,0.00000000002910383046,0.00000000001455191523,0.00000000000727595761,0.00000000000363797881,0.00000000000181898940,0.00000000000090949470,0.00000000000045474735,0.00000000000022737368,0.00000000000011368684,0.00000000000005684342,0.00000000000002842171,0.00000000000001421085,0.00000000000000710543,0.00000000000000355271,0.00000000000000177636,0.00000000000000088818,0.00000000000000044409,0.00000000000000022204,0.00000000000000011102,0.00000000000000005551,0.00000000000000002776,0.00000000000000001388,0.00000000000000000694,0.00000000000000000347,0.00000000000000000173,0.00000000000000000087,0.00000000000000000043,0.00000000000000000022,0.00000000000000000011];

x = xi;
y = yi;
t = 0;
if mi
    t = ti;
else
    t = 0;
end
for i = 1:1:20
    sigma = 0;
    if mi
        if t < 0
            sigma = -1;
        else
            sigma = 1;
        end
    else
        if y < 0
            sigma = 1;
        else
            sigma = -1;
        end
    end
    xs = x * sigma * 2^(-(i-1));
    ys = y * sigma * 2^(-(i-1));
    x = x - ys;
    y = y + xs;
    t = t - sigma * cordic_phase(i);
end
xo = x;
yo = y;
to = t;
end
